simulink model "IDriver"  (R2018a)
settings: Solver=FixedStepDiscrete  StartTime=0.0  StopTime=10.0  FixedStep=0.01  RelTol=1e-3
settings Model: Creator=zhoutinglin  LastModifiedBy=zhoutinglin
settings DataIOCC: SaveOutput=off  SignalLogging=off  DSMLogging=off  SaveTime=off
settings OptimizationCC: DefaultParameterBehavior=Inlined  EnhancedBackFolding=on  PassReuseOutputArgsAs=Individual arguments  OptimizeBlockOrder=speed  DifferentSizesBufferReuse=on  OptimizationCustomize=off
settings DebuggingCC: ParameterTunabilityLossMsg=error
settings SFSimCC: MATLABDynamicMemAlloc=off
settings RTWCC: SystemTargetFile=ert.tlc  GenCodeOnly=on  TemplateMakefile=ert_default_tmf  GenerateReport=on  IncludeHyperlinkInReport=on  LaunchReport=on  GenerateTraceInfo=on  GenerateTraceReport=on  GenerateTraceReportSl=on  GenerateTraceReportSf=on  GenerateTraceReportEml=on
settings CodeAppCC: ForceParamTrailComments=on  IgnoreCustomStorageClasses=off  OperatorAnnotations=on  SimulinkDataObjDesc=on  SFDataObjDesc=on  InsertBlockDesc=on
settings ERTTargetCC: TargetLangStandard=C99 (ISO)  GenerateSampleERTMain=on  SupportNonInlinedSFcns=on  InlinedParameterPlacement=NonHierarchical  ERTCustomFileTemplate=example_file_process.tlc

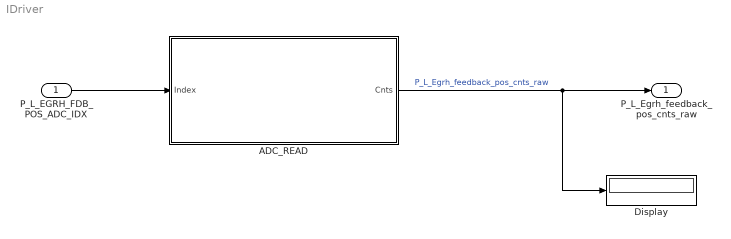
== system IDriver ==
  P_L_EGRH_FDB_POS_ADC_IDX : Inport
  ADC_READ : Subsystem  Variant=on  mask(ADC_Read){num_bits=10}
      mask prompts: num_bits "ADC counter accuracy(number of bits)"
      mask help: Variant Subsystem, used for Code Gen and Simulation.
      mask init:
      | num_bits_str=get_param(gcb,'num_bits');
      | num_bits_12_used=strcmp(num_bits_str,'12');
      | if num_bits_12_used
      |    set_param([gcb,'/ForSimulation/num_bits_12_used'],'Value','true');
      | else
      |    set_param([gcb,'/ForSimulation/num_bits_12_used'],'Value','false');
      | end
      | 
      | linesH = get(gcbh, 'LineHandles');
      | if  linesH.Inport(1) ~= -1
      |     srcblock = get(linesH.Inport(1), 'SrcBlockHandle');
      |     port_name = get(srcblock, 'Name');
      | else
      |     port_name = 'XXX';
      | end
      | % disp(name);
      | %P_L_ADC_RD_10BITS_V1_EGRH_FDB_POS()
      | driver_name=erase(erase(port_name,'P_L_'),'_ADC_IDX');
      | % disp(driver_name);
      | full_dirver_name=['P_L_ADC_RD_' num_bits_str 'BITS_V1_' driver_name];
      | % disp(full_dirver_name);
      | full_driver_name_unicode=unicode2native(full_dirver_name);
      | set_param([gcb,'/CodegenSFun/AD_Read_SFun'],'Parameters','full_driver_name_unicode');
      mask TypeOptions num_bits: 10 | 12
      mask Display:
      | fprintf(['Analog\nInput\nRead']);
      | % text(0.85, 0.9, '(v1)')
  Display : Display
  P_L_Egrh_feedback_pos_cnts_raw : Outport
  wires:
  ADC_READ/1(Cnts) -> Display/1, P_L_Egrh_feedback_pos_cnts_raw/1  "P_L_Egrh_feedback_pos_cnts_raw"
  P_L_EGRH_FDB_POS_ADC_IDX/1 -> ADC_READ/1(Index)

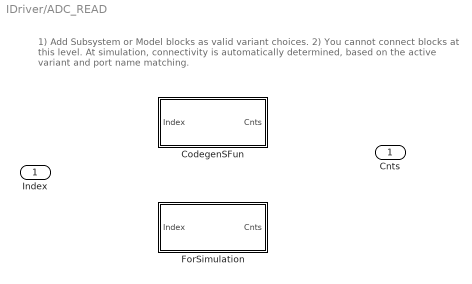
== system IDriver/ADC_READ ==
  note: 1) Add Subsystem or Model blocks as valid variant choices.
      | 2) You cannot connect blocks at this level. At simulation, connectivity is automatically
      | determined, based on the active variant and port name matching.
  Index : Inport
  CodegenSFun : Subsystem  VariantControl=varCodegenChoosed
  ForSimulation : Subsystem  VariantControl=(default)
  Cnts : Outport

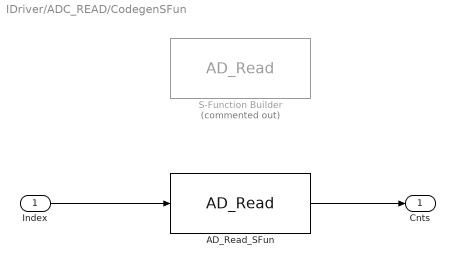
== system IDriver/ADC_READ/CodegenSFun ==
  Index : Inport
  AD_Read_SFun : S-Function  FunctionName=AD_Read  Parameters=full_driver_name_unicode  SFunctionDeploymentMode=off  EnableBusSupport=off
  S-Function Builder : S-Function  Commented=on  InitFcn=try, set_param(gcb,'FunctionName','AD_Read'), end  FunctionName=AD_Read  Parameters=uint8(1)  SFunctionModules=AD_Read_wrapper  SFunctionDeploymentMode=off  EnableBusSupport=off  mask(S-Function Builder){}
      mask help: Simulink:masks:SFunctionBuilder_MD
      mask init:
      | val = [[.9  0.75 0.75 1 1 .9 .9 1]',[1 1 0.75 0.75 .9 .9 1 .9]'];try , sys = get_param(gcb,'SfunBuilderFcnName');if isempty(sys), sys = get_param(gcb,'FunctionName'); end,catch, sys = get_param(gcb,'FunctionName'); end
      settings: CopyFcn=set_param(gcbh,'LinkStatus','none')  PreSaveFcn=try, set_param(gcb,'FunctionName','AD_Read'), end  OpenFcn=sfunctionwizard(gcbh)
      mask Display: plot(val(:,1),val(:,2)),disp(sys), port_label('input',1,'Index'), port_label('output',1,'Cnts')
  Cnts : Outport
  wires:
  Index/1 -> AD_Read_SFun/1
  AD_Read_SFun/1 -> Cnts/1

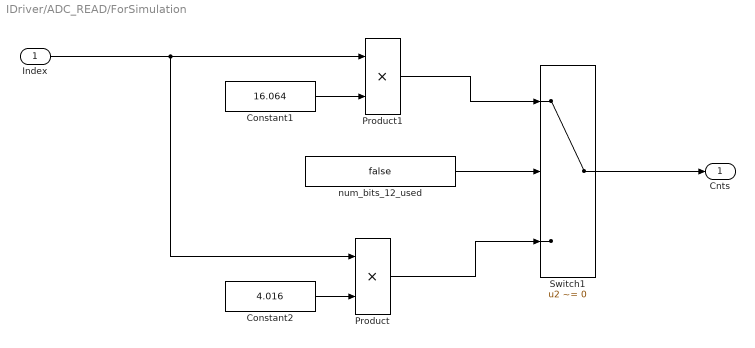
== system IDriver/ADC_READ/ForSimulation ==
  Index : Inport
  Constant1 : Constant  Value=16.064  OutDataTypeStr=fixdt(1,32,2^-24,0)
  Constant2 : Constant  Value=4.016  OutDataTypeStr=fixdt(1,32,2^-24,0)
  Product : Product  OutDataTypeStr=uint16
  Product1 : Product  OutDataTypeStr=uint16
  Switch1 : Switch  Criteria=u2 ~= 0  InputSameDT=on
  num_bits_12_used : Constant  Value=false  OutDataTypeStr=boolean
  Cnts : Outport
  wires:
  num_bits_12_used/1 -> Switch1/2
  Product1/1 -> Switch1/1
  Switch1/1 -> Cnts/1
  Product/1 -> Switch1/3
  Index/1 -> Product/1, Product1/1
  Constant1/1 -> Product1/2
  Constant2/1 -> Product/2
